simulink model "model2a"  (R2017a)
settings: Solver=VariableStepAuto  StartTime=0.0  StopTime=.5  RelTol=1e-3
undefined symbols (not defined in the file): K
settings Model: Creator=vjdixit2  LastModifiedBy=vjdixit2

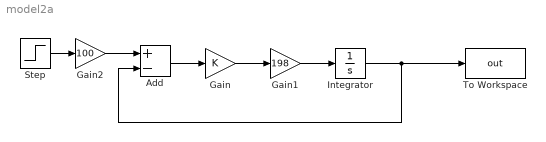
== system model2a ==
  Add : Sum  Inputs=+-
  Gain : Gain  Gain=K
  Gain1 : Gain  Gain=198
  Gain2 : Gain  Gain=100
  Integrator : Integrator
  Step : Step  Time=0  SampleTime=0
  To Workspace : ToWorkspace  VariableName=out  SampleTime=-1
  wires:
  Step/1 -> Gain2/1
  Add/1 -> Gain/1
  Gain/1 -> Gain1/1
  Gain1/1 -> Integrator/1
  Integrator/1 -> Add/2, To Workspace/1
  Gain2/1 -> Add/1
